simulink model "lab5"  (Simulink 8.5)
settings: Solver=ode23tb  StartTime=0.0  StopTime=2.5  RelTol=1e-3
libraries: powerlib x5, lib_Timer_Counter x1
settings Model: Creator=Sarmad  LastModifiedBy=Enigma
settings SolverCC: SolverResetMethod=Robust
settings DebuggingCC: SolverPrmCheckMsg=warning  FcnCallInpInsideContextMsg=UseLocalSettings

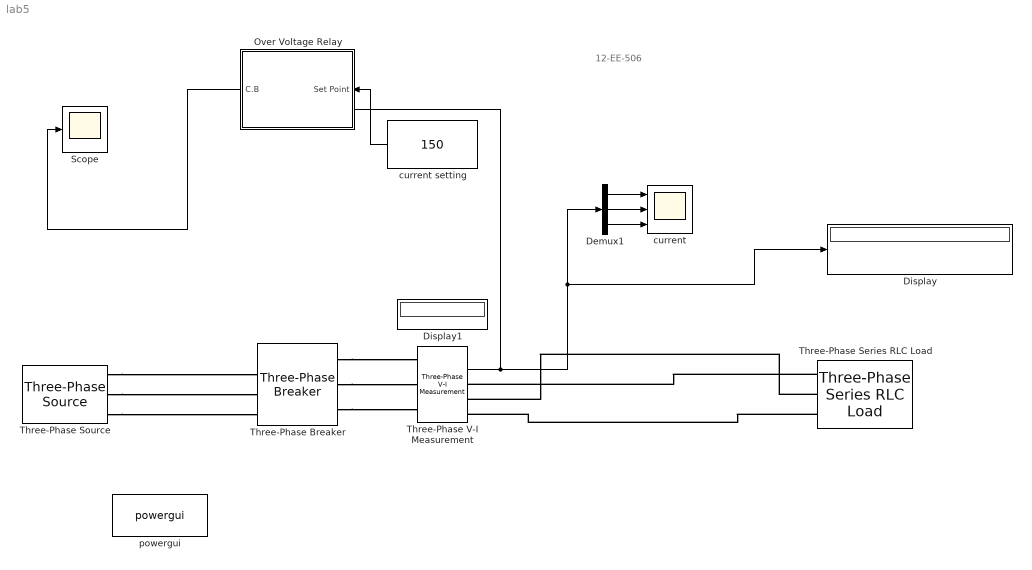
== system lab5 ==
  note: 12-EE-506
  Demux1 : Demux  Outputs=3
  Display : Display
  Display1 : Display
  Over Voltage Relay : Subsystem
  Scope : Scope
      settings: TimeRange=0.35  YMin=0  YMax=1  SaveName=ScopeData2
  Three-Phase Series RLC Load : powerlib/Elements/Three-Phase Series RLC Load  LConnTagsString=A|B|C  Configuration=Y (grounded)  NominalVoltage=220  NominalFrequency=50  ActivePower=100e6  InductivePower=10e4  CapacitivePower=0  Measurements=None  LoadType=constant Z
  Three-Phase V-I Measurement : powerlib/Measurements/Three-Phase V-I Measurement  VoltageMeasurement=phase-to-phase  SetLabelV=off  LabelV=Vabc  Vpu=off  VpuLL=off  CurrentMeasurement=yes  SetLabelI=off  LabelI=Iabc  Ipu=off  Pbase=100e6  Vbase=500e3  OutputType=Complex  PhasorSimulation=off  PSBequivalent=0
  Three-Phase Breaker : powerlib/Elements/Three-Phase Breaker  InitialState=closed  SwitchA=on  SwitchB=on  SwitchC=on  SwitchTimes="[4/60  10/60]"  External=on  BreakerResistance=0.001  SnubberResistance=1e6  SnubberCapacitance=inf  Measurements=None
  Three-Phase Source : powerlib/Electrical Sources/Three-Phase Source  Voltage=220  PhaseAngle=0  Frequency=50  InternalConnection=Yg  SpecifyImpedance=on  Resistance=0.8929  Inductance=16.58e-3  ShortCircuitLevel=500e6  BaseVoltage=11e3  XRratio=7  BusType=swing  Pref=0  Qref=0  Qmin=-inf  Qmax=inf
  current : Scope  NumInputPorts=3
      settings: TimeRange=0.25  YMin=-30000~-5~-5  YMax=30000~5~5  SampleInput=on
  current setting : Constant  Value=150
  powergui : powerlib/powergui  Priority=1  SimulationMode=Discrete  SolverType=Tustin/Backward Euler (TBE)  SampleTime=5e-005  frequency=60  SPID=off  DisableSnubberDevices=off  DisableRonSwitches=off  DisableVfSwitches=off  SwTol=0  DisplayEquations=off  Interpol=off  methode=off  Ts=0  FunctionMessages=off  echomessages=off  HookPort=off  EnableUseOfTLC=off  x0status=blocks  frequencyindice=0  Pbase=100e6  ErrMax=1e-4  Iterations=50  UnitsV=kV  UnitsW=MW  buscounter=0  RestoreLinks=warning  ResistiveCurrentMeasurement=off  Frange=[0:2:500]  Ylog=off  Xlog=on  ShowGrid=off  save=off  variable=ZData  structure=0  ZoomFFT=on  StartTime=0.0  cycles=1  DisplayStyle=1  fundamental=60  FreqAxis=off  MaxFrequency=1000  frequencyindicesteady=1  RmsSteady=2  display=off
  wires:
  Three-Phase V-I Measurement/2 -> Demux1/1, Display/1
  current setting/1 -> Over Voltage Relay/1(Set Point)
  Demux1/1 -> current/1
  Demux1/2 -> current/2
  Demux1/3 -> current/3
  Over Voltage Relay/1(C.B) -> Scope/1
  connections:
  Three-Phase Source/RConn1 -- Three-Phase Breaker/LConn1
  Three-Phase Source/RConn2 -- Three-Phase Breaker/LConn2
  Three-Phase Source/RConn3 -- Three-Phase Breaker/LConn3
  Three-Phase Breaker/RConn1 -- Three-Phase V-I Measurement/LConn1
  Three-Phase Breaker/RConn2 -- Three-Phase V-I Measurement/LConn2
  Three-Phase Breaker/RConn3 -- Three-Phase V-I Measurement/LConn3
  Three-Phase Series RLC Load/LConn3 -- Three-Phase V-I Measurement/RConn3
  Three-Phase Series RLC Load/LConn2 -- Three-Phase V-I Measurement/RConn2
  Three-Phase Series RLC Load/LConn1 -- Three-Phase V-I Measurement/RConn1

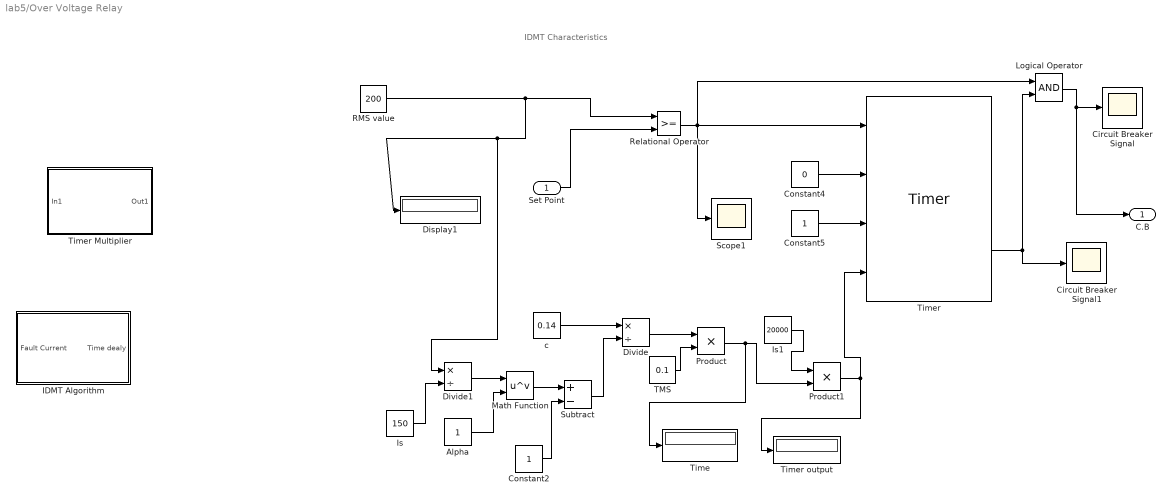
== system lab5/Over Voltage Relay ==
  note: IDMT Characteristics
  Set Point : Inport  OutDataTypeStr=double
  Alpha : Constant  OutDataTypeStr=double
  Circuit Breaker Signal : Scope
      settings: TimeRange=0.35  YMin=1  YMax=1  SaveName=ScopeData6
  Circuit Breaker Signal1 : Scope
      settings: TimeRange=0.35  YMin=1  YMax=1
  Constant2 : Constant  OutDataTypeStr=double
  Constant4 : Constant  Value=0  OutDataTypeStr=double
  Constant5 : Constant  OutDataTypeStr=double
  Display1 : Display
  Divide : Product  Inputs=*/
  Divide1 : Product  Inputs=*/
  IDMT Algorithm : Subsystem
  Is : Constant  Value=150  OutDataTypeStr=double
  Is1 : Constant  Value=20000  OutDataTypeStr=double
  Logical Operator : Logic  AllPortsSameDT=off  OutDataTypeStr=boolean
  Math Function : Math  Operator=pow  SaturateOnIntegerOverflow=on
  Product : Product
  Product1 : Product
  RMS value : Constant  Value=200  OutDataTypeStr=double
  Relational Operator : RelationalOperator  OutDataTypeStr=boolean
  Scope1 : Scope
      settings: TimeRange=0.35  YMin=0  YMax=1  SaveName=ScopeData4
  Subtract : Sum  Inputs=+-
  TMS : Constant  Value=0.1  OutDataTypeStr=double
  Time : Display
  Timer : lib_Timer_Counter/Timer
  Timer Multiplier : Subsystem
  Timer output : Display
  c : Constant  Value=0.14  OutDataTypeStr=double
  C.B : Outport
  wires:
  Constant4/1 -> Timer/2
  Constant5/1 -> Timer/3
  Timer/2 -> Circuit Breaker Signal1/1, Logical Operator/2
  Set Point/1 -> Relational Operator/2
  Logical Operator/1 -> Circuit Breaker Signal/1, C.B/1
  Relational Operator/1 -> Timer/1, Scope1/1, Logical Operator/1
  c/1 -> Divide/1
  Subtract/1 -> Divide/2
  Constant2/1 -> Subtract/2
  Math Function/1 -> Subtract/1
  Divide1/1 -> Math Function/1
  Divide/1 -> Product/1
  RMS value/1 -> Divide1/1, Display1/1, Relational Operator/1
  Is/1 -> Divide1/2
  Alpha/1 -> Math Function/2
  TMS/1 -> Product/2
  Product1/1 -> Timer output/1, Timer/4
  Product/1 -> Time/1, Product1/2
  Is1/1 -> Product1/1

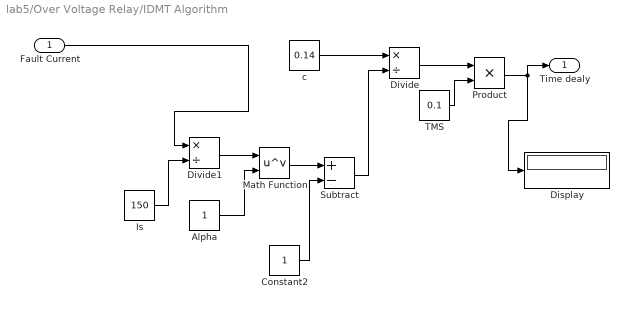
== system lab5/Over Voltage Relay/IDMT Algorithm ==
  Fault Current : Inport
  Alpha : Constant  OutDataTypeStr=double
  Constant2 : Constant  OutDataTypeStr=double
  Display : Display
  Divide : Product  Inputs=*/
  Divide1 : Product  Inputs=*/
  Is : Constant  Value=150  OutDataTypeStr=double
  Math Function : Math  Operator=pow  SaturateOnIntegerOverflow=on
  Product : Product
  Subtract : Sum  Inputs=+-
  TMS : Constant  Value=0.1  OutDataTypeStr=double
  c : Constant  Value=0.14  OutDataTypeStr=double
  Time dealy : Outport
  wires:
  c/1 -> Divide/1
  Subtract/1 -> Divide/2
  Constant2/1 -> Subtract/2
  Math Function/1 -> Subtract/1
  Divide1/1 -> Math Function/1
  Divide/1 -> Product/1
  Fault Current/1 -> Divide1/1
  Is/1 -> Divide1/2
  Alpha/1 -> Math Function/2
  TMS/1 -> Product/2
  Product/1 -> Display/1, Time dealy/1

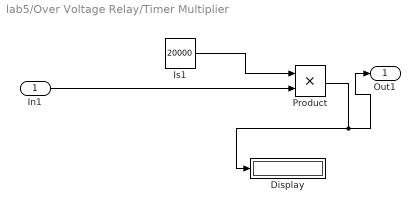
== system lab5/Over Voltage Relay/Timer Multiplier ==
  In1 : Inport
  Display : Display
  Is1 : Constant  Value=20000  OutDataTypeStr=double
  Product : Product
  Out1 : Outport
  wires:
  Product/1 -> Out1/1, Display/1
  In1/1 -> Product/2
  Is1/1 -> Product/1
